simulink model "sin_cos"  (R2019a)
settings: Solver=VariableStepAuto  StartTime=0.0  StopTime=10.0  RelTol=1e-3
settings Model: Creator=Egypt_Laptop  LastModifiedBy=Egypt_Laptop

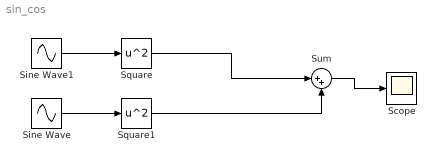
== system sin_cos ==
  Scope : Scope
  Sine Wave : Sin  Phase=pi/2  SampleTime=0
  Sine Wave1 : Sin  SampleTime=0
  Square : Math  Operator=square  SaturateOnIntegerOverflow=on
  Square1 : Math  Operator=square  SaturateOnIntegerOverflow=on
  Sum : Sum  Inputs=|++
  wires:
  Sine Wave1/1 -> Square/1
  Sine Wave/1 -> Square1/1
  Square/1 -> Sum/1
  Square1/1 -> Sum/2
  Sum/1 -> Scope/1
